simulink model "lab2part1"  (R2020b)
settings: Solver=VariableStepAuto  StartTime=0.0  StopTime=3  RelTol=1e-3
settings Model: Creator=Nikita  LastModifiedBy=Nikita

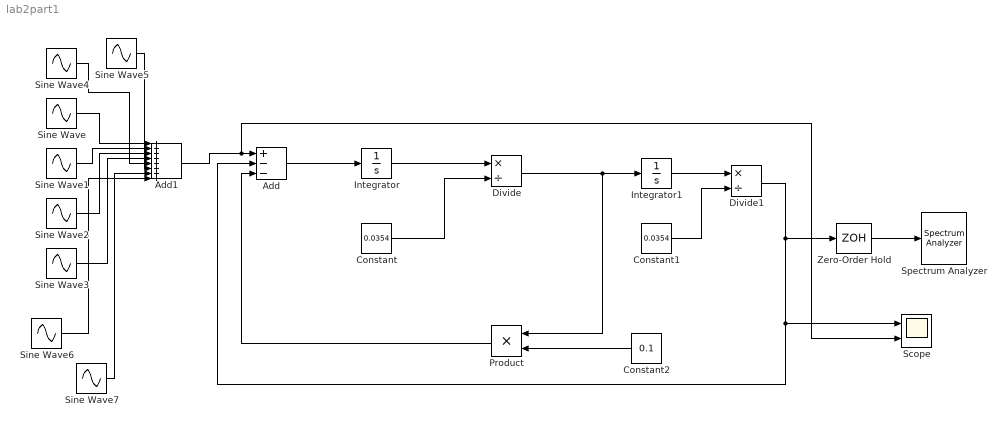
== system lab2part1 ==
  Add : Sum  Inputs=+--
  Add1 : Sum  Inputs=++++++++
  Constant : Constant  Value=0.0354
  Constant1 : Constant  Value=0.0354
  Constant2 : Constant  Value=0.1
  Divide : Product  Inputs=*/
  Divide1 : Product  Inputs=*/
  Integrator : Integrator
  Integrator1 : Integrator
  Product : Product
  Scope : Scope  NumInputPorts=2
  Sine Wave : Sin  Amplitude=4/(pi*1)  Frequency=64*pi  SampleTime=0
  Sine Wave1 : Sin  Amplitude=4/(pi*3)  Frequency=192*pi  SampleTime=0
  Sine Wave2 : Sin  Amplitude=4/(pi*5)  Frequency=320*pi  SampleTime=0
  Sine Wave3 : Sin  Amplitude=4/(pi*7)  Frequency=448*pi  SampleTime=0
  Sine Wave4 : Sin  Amplitude=4/(pi*11)  Frequency=704*pi  SampleTime=0
  Sine Wave5 : Sin  Amplitude=4/(pi*9)  Frequency=576*pi  SampleTime=0
  Sine Wave6 : Sin  Amplitude=4/(pi*13)  Frequency=64*pi*13  SampleTime=0
  Sine Wave7 : Sin  Amplitude=4/(pi*15)  Frequency=64*pi*15  SampleTime=0
  Spectrum Analyzer : SpectrumAnalyzer
  Zero-Order Hold : ZeroOrderHold  SampleTime=2^-10
  wires:
  Constant/1 -> Divide/2
  Divide/1 -> Integrator1/1, Product/1
  Constant1/1 -> Divide1/2
  Constant2/1 -> Product/2
  Product/1 -> Add/3
  Zero-Order Hold/1 -> Spectrum Analyzer/1
  Add/1 -> Integrator/1
  Integrator/1 -> Divide/1
  Integrator1/1 -> Divide1/1
  Divide1/1 -> Zero-Order Hold/1, Add/2, Scope/1
  Add1/1 -> Scope/2, Add/1
  Sine Wave3/1 -> Add1/4
  Sine Wave1/1 -> Add1/2
  Sine Wave7/1 -> Add1/7
  Sine Wave/1 -> Add1/1
  Sine Wave6/1 -> Add1/8
  Sine Wave2/1 -> Add1/3
  Sine Wave5/1 -> Add1/6
  Sine Wave4/1 -> Add1/5
